simulink model "Fig515"  (R2014b)
settings: Solver=ode3  StartTime=0.0  StopTime=.128  FixedStep=1e-3  RelTol=1e-3
libraries: commseqgen2 x2, simulink_extras x1
settings Model: Creator=Silage  LastModifiedBy=Silage

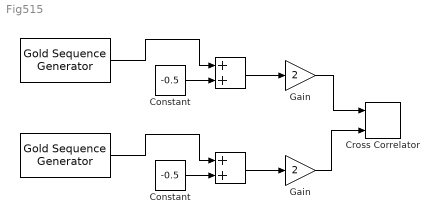
== system Fig515 ==
  "  " : commseqgen2/Gold Sequence Generator  genPoly1=[1 0 0 1 0 1]  iniState1=[1 1 1 0 1]  genPoly2=[1 1 1 1 0 1]  iniState2=[1 0 0 0 1]  index=0  shift=0  outVarSiz=off  maxOutSizeMode=Dialog parameter  maxOutSize=[10 1]  ts=1e-3  frameBased=off  sampPerFrame=1  reset=off  outDataType=double
  "    " : Sum
  "     " : commseqgen2/Gold Sequence Generator  genPoly1=[1 0 0 1 0 1]  iniState1=[1 0 1 0 1]  genPoly2=[1 1 1 1 0 1]  iniState2=[1 1 1 0 0]  index=0  shift=0  outVarSiz=off  maxOutSizeMode=Dialog parameter  maxOutSize=[10 1]  ts=1e-3  frameBased=off  sampPerFrame=1  reset=off  outDataType=double
  "       " : Sum
  " Constant " : Constant  Value=-0.5
  " Gain " : Gain  Gain=2
  Constant : Constant  Value=-0.5
  Cross Correlator : simulink_extras/Additional Sinks/Cross Correlator  npts=128  HowOften=128  sampleT=1e-3
  Gain : Gain  Gain=2
  wires:
  "  "/1 -> "    "/1
  Constant/1 -> "    "/2
  "    "/1 -> Gain/1
  Gain/1 -> Cross Correlator/1
  "     "/1 -> "       "/1
  " Constant "/1 -> "       "/2
  "       "/1 -> " Gain "/1
  " Gain "/1 -> Cross Correlator/2
